simulink model "lab4_mc"  (R2023a)
settings: Solver=FixedStepAuto  StartTime=0.0  StopTime=inf  FixedStep=0.001  RelTol=1e-3
undefined symbols (not defined in the file): CR, LF
libraries: instrumentseriallib x3
settings Model: Creator=shume  LastModifiedBy=shume

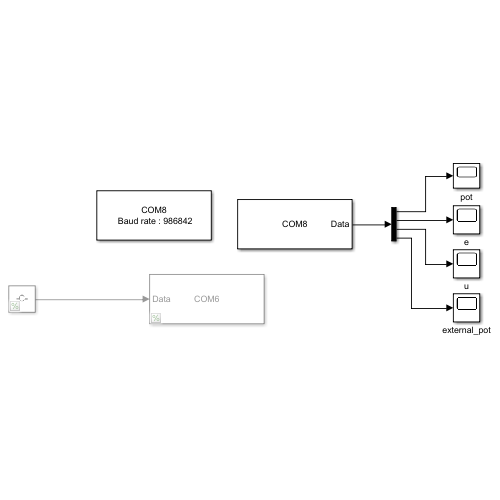
[thumbnail: Simulink's stored preview of the top-level diagram]
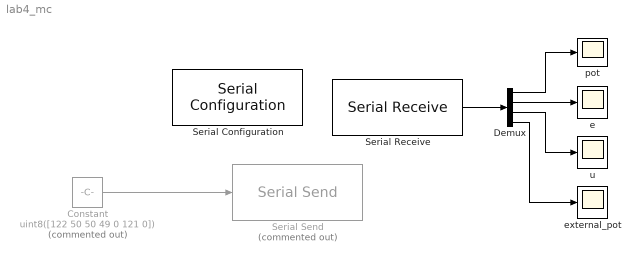
== system lab4_mc ==
  Constant : Constant  Commented=on  Value=uint8([122 50 50 49 0 121 0])
  Demux : Demux
  Serial Configuration : instrumentseriallib/Serial Configuration  Priority=-200000  PortSel=COM8  Port=COM8  ComPort=COM8  BaudRate=986842  DataBits=8  Parity=none  StopBits=1  ByteOrder=little-endian  FlowControl=none  Timeout=20  SimulateUsing=Interpreted execution  BlockInModel=on  aMode=1
  Serial Receive : instrumentseriallib/Serial Receive  Priority=1  PortSel=COM8  Port=COM8  ComPort=COM8  DataType=uint32  SaveDataType=uint8  ToggleHeader=on  Header=[0xAA 0xAA 0xAA 0xAA]  ToggleTerminator=off  Terminator=<none>  CustomTerminator=[]  InputFormat=Column major  ToggleDataSize=on  DataSize=[4 1]  EnableBlockingMode=on  ActionDataUnavailable=Output last received value  ActionWhenDataUnavailable=Output last received value  CustomValue=0  SampleTime=-1  SimulateUsing=Interpreted execution  BlockInModel=on  aMode=1
  Serial Send : instrumentseriallib/Serial Send  Priority=1  Commented=on  PortSel=COM6  Port=COM6  ComPort=COM6  Header=[]  Terminator=CR/LF ('\r\n')  CustomTerminator=[]  EnableBlockingMode=on  SimulateUsing=Interpreted execution  BlockInModel=on  aMode=1
  e : Scope
  external_pot : Scope
  pot : Scope
  u : Scope
  wires:
  Constant/1 -> Serial Send/1
  Serial Receive/1 -> Demux/1
  Demux/2 -> e/1
  Demux/1 -> pot/1
  Demux/3 -> u/1
  Demux/4 -> external_pot/1
